simulink model "TransferFnc"  (R2018b)
settings: Solver=VariableStepAuto  StartTime=0.0  StopTime=6  RelTol=1e-3
settings Model: Creator=franboonham  LastModifiedBy=franboonham
settings DataIOCC: ReturnWorkspaceOutputs=on

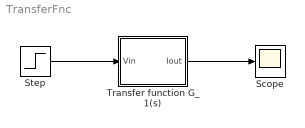
== system TransferFnc ==
  Scope : Scope
  Step : Step  SampleTime=0
  Transfer function G_1(s) : Subsystem
      mask init:
      | L = 0.5*10^-3;
      | R = 75;
  wires:
  Step/1 -> Transfer function G_1(s)/1(Vin)
  Transfer function G_1(s)/1(Iout) -> Scope/1

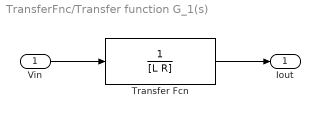
== system TransferFnc/Transfer function G_1(s) ==
  Vin : Inport
  Transfer Fcn : TransferFcn  Denominator=[L R]
  Iout : Outport
  wires:
  Vin/1 -> Transfer Fcn/1
  Transfer Fcn/1 -> Iout/1
